simulink model "assignment_1"  (R2023b)
settings: Solver=ode3  StartTime=0.0  StopTime=Tmdl  FixedStep=To/100  RelTol=1e-3
values from neighbouring files (symbols this model uses):
  ob =     [data.mat]
undefined symbols (not defined in the file or in its folder): k_sensor, spl, T_sensor, To
libraries: fl_lib x33, nesl_utility x27
settings Model: Creator=deniskirbaba  LastModifiedBy=deniskirbaba

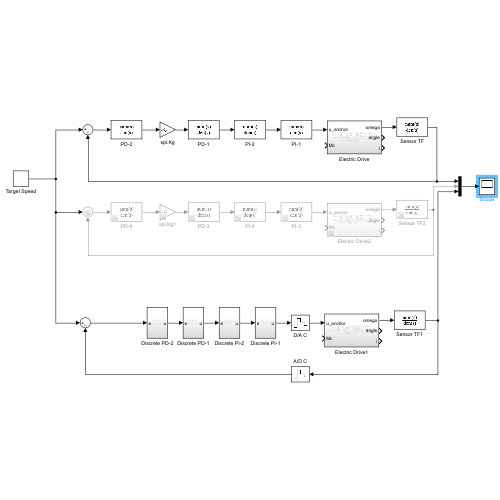
[thumbnail: Simulink's stored preview of the top-level diagram]
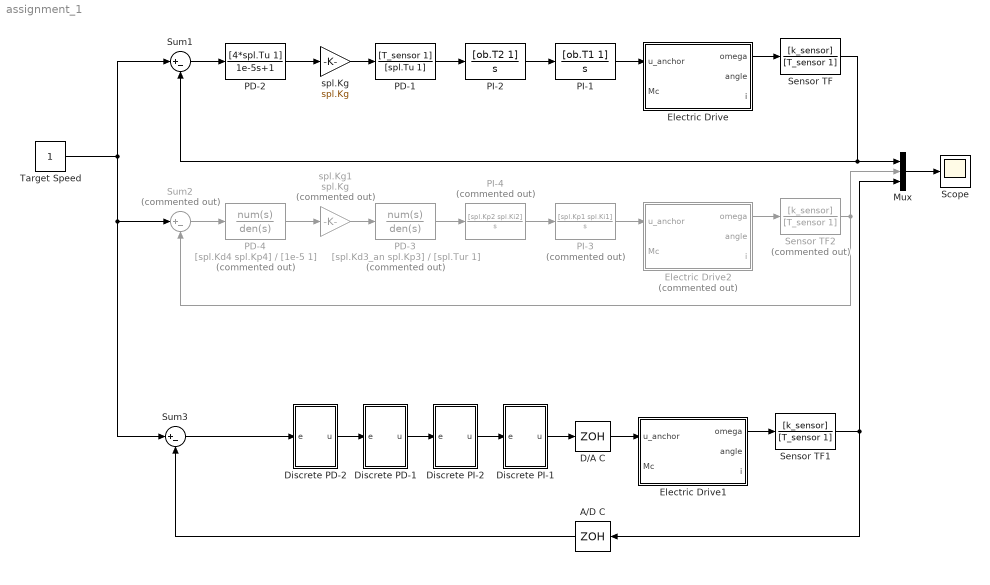
== system assignment_1 ==
  A/D C : ZeroOrderHold  SampleTime=To
  D/A C : ZeroOrderHold  SampleTime=To
  Discrete PD-1 : Subsystem
  Discrete PD-2 : Subsystem
  Discrete PI-1 : Subsystem
  Discrete PI-2 : Subsystem
  Electric Drive : Subsystem
  Electric Drive1 : Subsystem
  Electric Drive2 : Subsystem  Commented=on
  Mux : Mux  Inputs=3
  PD-1 : TransferFcn  Numerator=[T_sensor 1]  Denominator=[spl.Tu 1]
  PD-2 : TransferFcn  Numerator=[4*spl.Tu 1]  Denominator=[1e-5 1]
  PD-3 : TransferFcn  Commented=on  Numerator=[spl.Kd3_an spl.Kp3]  Denominator=[spl.Tur 1]
  PD-4 : TransferFcn  Commented=on  Numerator=[spl.Kd4 spl.Kp4]  Denominator=[1e-5 1]
  PI-1 : TransferFcn  Numerator=[ob.T1 1]  Denominator=[1 0]
  PI-2 : TransferFcn  Numerator=[ob.T2 1]  Denominator=[1 0]
  PI-3 : TransferFcn  Commented=on  Numerator=[spl.Kp1 spl.Ki1]  Denominator=[1 0]
  PI-4 : TransferFcn  Commented=on  Numerator=[spl.Kp2 spl.Ki2]  Denominator=[1 0]
  Scope : Scope
  Sensor TF : TransferFcn  Numerator=[k_sensor]  Denominator=[T_sensor 1]
  Sensor TF1 : TransferFcn  Numerator=[k_sensor]  Denominator=[T_sensor 1]
  Sensor TF2 : TransferFcn  Commented=on  Numerator=[k_sensor]  Denominator=[T_sensor 1]
  Sum1 : Sum  Inputs=|+-
  Sum2 : Sum  Commented=on  Inputs=|+-
  Sum3 : Sum  Inputs=|+-
  Target Speed : Constant
  spl.Kg : Gain  Gain=spl.Kg
  spl.Kg1 : Gain  Commented=on  Gain=spl.Kg
  wires:
  Electric Drive1/1(omega) -> Sensor TF1/1
  Mux/1 -> Scope/1
  D/A C/1 -> Electric Drive1/1(u_anchor)
  A/D C/1 -> Sum3/2
  Electric Drive/1(omega) -> Sensor TF/1
  Sum3/1 -> Discrete PD-2/1(e)
  Sum1/1 -> PD-2/1
  Discrete PD-1/1(u) -> Discrete PI-2/1(e)
  Sensor TF/1 -> Sum1/2, Mux/1
  Sensor TF1/1 -> A/D C/1, Mux/3
  PI-1/1 -> Electric Drive/1(u_anchor)
  PD-2/1 -> spl.Kg/1
  PI-2/1 -> PI-1/1
  PD-1/1 -> PI-2/1
  spl.Kg/1 -> PD-1/1
  Discrete PI-1/1(u) -> D/A C/1
  Discrete PI-2/1(u) -> Discrete PI-1/1(e)
  Discrete PD-2/1(u) -> Discrete PD-1/1(e)
  spl.Kg1/1 -> PD-3/1
  Electric Drive2/1(omega) -> Sensor TF2/1
  PD-3/1 -> PI-4/1
  PI-4/1 -> PI-3/1
  PD-4/1 -> spl.Kg1/1
  PI-3/1 -> Electric Drive2/1(u_anchor)
  Sum2/1 -> PD-4/1
  Target Speed/1 -> Sum1/1, Sum3/1, Sum2/1
  Sensor TF2/1 -> Sum2/2, Mux/2

== system assignment_1/Discrete PD-1 ==
  e : Inport
  D-regulator2 : Subsystem
  Sum4 : Sum  Inputs=++|
  spl.Kd3 : Gain  Gain=spl.Kd3
  spl.Kp3 : Gain  Gain=spl.Kp3
  u : Outport
  wires:
  e/1 -> spl.Kd3/1, spl.Kp3/1
  spl.Kd3/1 -> D-regulator2/1(e)
  spl.Kp3/1 -> Sum4/1
  D-regulator2/1(u) -> Sum4/2
  Sum4/1 -> u/1

== system assignment_1/Discrete PD-2 ==
  e : Inport
  D-regulator2 : Subsystem
  Sum4 : Sum  Inputs=++|
  spl.Kd4 : Gain  Gain=spl.Kd4
  spl.Kp4 : Gain  Gain=spl.Kp4
  u : Outport
  wires:
  e/1 -> spl.Kd4/1, spl.Kp4/1
  spl.Kd4/1 -> D-regulator2/1(e)
  spl.Kp4/1 -> Sum4/1
  D-regulator2/1(u) -> Sum4/2
  Sum4/1 -> u/1

== system assignment_1/Discrete PI-1 ==
  e : Inport
  Sum2 : Sum  Inputs=|++
  i trap : Subsystem
  spl.Ki1 : Gain  Gain=spl.Ki1
  spl.Kp1 : Gain  Gain=spl.Kp1
  u : Outport
  wires:
  e/1 -> spl.Ki1/1, spl.Kp1/1
  spl.Kp1/1 -> Sum2/1
  Sum2/1 -> u/1
  i trap/1(u) -> Sum2/2
  spl.Ki1/1 -> i trap/1(e)

== system assignment_1/Discrete PI-2 ==
  e : Inport
  Sum2 : Sum  Inputs=|++
  i trap : Subsystem
  spl.Ki2 : Gain  Gain=spl.Ki2
  spl.Kp2 : Gain  Gain=spl.Kp2
  u : Outport
  wires:
  e/1 -> spl.Ki2/1, spl.Kp2/1
  spl.Kp2/1 -> Sum2/1
  Sum2/1 -> u/1
  i trap/1(u) -> Sum2/2
  spl.Ki2/1 -> i trap/1(e)

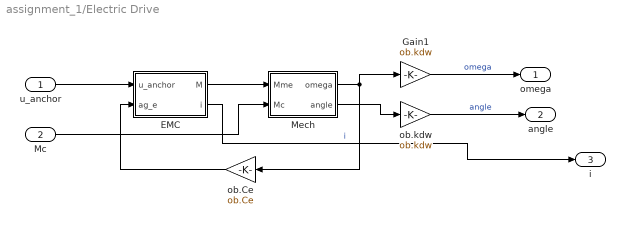
== system assignment_1/Electric Drive ==
  u_anchor : Inport
  Mc : Inport  Port=2
  EMC : Subsystem
  Gain1 : Gain  Gain=ob.kdw
  Mech : Subsystem
  ob.Ce : Gain  Gain=ob.Ce
  ob.kdw : Gain  Gain=ob.kdw
  omega : Outport
  angle : Outport  Port=2
  i : Outport  Port=3
  wires:
  Mech/1(omega) -> ob.Ce/1, Gain1/1
  Mc/1 -> Mech/2(Mc)
  Gain1/1 -> omega/1  "omega"
  EMC/1(M) -> Mech/1(Mme)
  ob.kdw/1 -> angle/1  "angle"
  Mech/2(angle) -> ob.kdw/1
  EMC/2(i) -> i/1  "i"
  ob.Ce/1 -> EMC/2(ag_e)
  u_anchor/1 -> EMC/1(u_anchor)

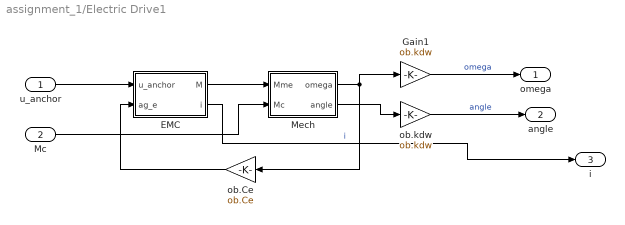
== system assignment_1/Electric Drive1 ==
  u_anchor : Inport
  Mc : Inport  Port=2
  EMC : Subsystem
  Gain1 : Gain  Gain=ob.kdw
  Mech : Subsystem
  ob.Ce : Gain  Gain=ob.Ce
  ob.kdw : Gain  Gain=ob.kdw
  omega : Outport
  angle : Outport  Port=2
  i : Outport  Port=3
  wires:
  Mech/1(omega) -> ob.Ce/1, Gain1/1
  Mc/1 -> Mech/2(Mc)
  Gain1/1 -> omega/1  "omega"
  EMC/1(M) -> Mech/1(Mme)
  ob.kdw/1 -> angle/1  "angle"
  Mech/2(angle) -> ob.kdw/1
  EMC/2(i) -> i/1  "i"
  ob.Ce/1 -> EMC/2(ag_e)
  u_anchor/1 -> EMC/1(u_anchor)

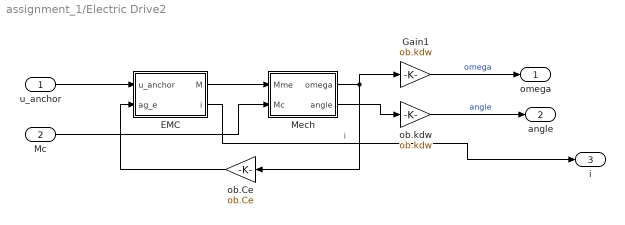
== system assignment_1/Electric Drive2 ==
  u_anchor : Inport
  Mc : Inport  Port=2
  EMC : Subsystem
  Gain1 : Gain  Gain=ob.kdw
  Mech : Subsystem
  ob.Ce : Gain  Gain=ob.Ce
  ob.kdw : Gain  Gain=ob.kdw
  omega : Outport
  angle : Outport  Port=2
  i : Outport  Port=3
  wires:
  Mech/1(omega) -> ob.Ce/1, Gain1/1
  Mc/1 -> Mech/2(Mc)
  Gain1/1 -> omega/1  "omega"
  EMC/1(M) -> Mech/1(Mme)
  ob.kdw/1 -> angle/1  "angle"
  Mech/2(angle) -> ob.kdw/1
  EMC/2(i) -> i/1  "i"
  ob.Ce/1 -> EMC/2(ag_e)
  u_anchor/1 -> EMC/1(u_anchor)

== system assignment_1/Discrete PD-1/D-regulator2 ==
  e : Inport
  Sum : Sum  Inputs=|+-
  Unit Delay : UnitDelay  SampleTime=To  HasFrameUpgradeWarning=on
  u : Outport
  wires:
  Unit Delay/1 -> Sum/2
  e/1 -> Unit Delay/1, Sum/1
  Sum/1 -> u/1

== system assignment_1/Discrete PD-2/D-regulator2 ==
  e : Inport
  Sum : Sum  Inputs=|+-
  Unit Delay : UnitDelay  SampleTime=To  HasFrameUpgradeWarning=on
  u : Outport
  wires:
  Unit Delay/1 -> Sum/2
  e/1 -> Unit Delay/1, Sum/1
  Sum/1 -> u/1

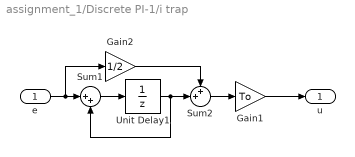
== system assignment_1/Discrete PI-1/i trap ==
  e : Inport
  Gain1 : Gain  Gain=To
  Gain2 : Gain  Gain=1/2
  Sum1 : Sum  Inputs=|++
  Sum2 : Sum  Inputs=++|
  Unit Delay1 : UnitDelay  SampleTime=To  HasFrameUpgradeWarning=on
  u : Outport
  wires:
  Unit Delay1/1 -> Sum2/2, Sum1/2
  Sum2/1 -> Gain1/1
  Gain2/1 -> Sum2/1
  Sum1/1 -> Unit Delay1/1
  e/1 -> Gain2/1, Sum1/1
  Gain1/1 -> u/1

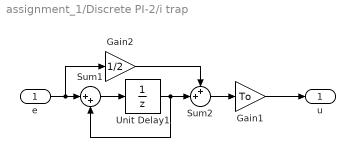
== system assignment_1/Discrete PI-2/i trap ==
  e : Inport
  Gain1 : Gain  Gain=To
  Gain2 : Gain  Gain=1/2
  Sum1 : Sum  Inputs=|++
  Sum2 : Sum  Inputs=++|
  Unit Delay1 : UnitDelay  SampleTime=To  HasFrameUpgradeWarning=on
  u : Outport
  wires:
  Unit Delay1/1 -> Sum2/2, Sum1/2
  Sum2/1 -> Gain1/1
  Gain2/1 -> Sum2/1
  Sum1/1 -> Unit Delay1/1
  e/1 -> Gain2/1, Sum1/1
  Gain1/1 -> u/1

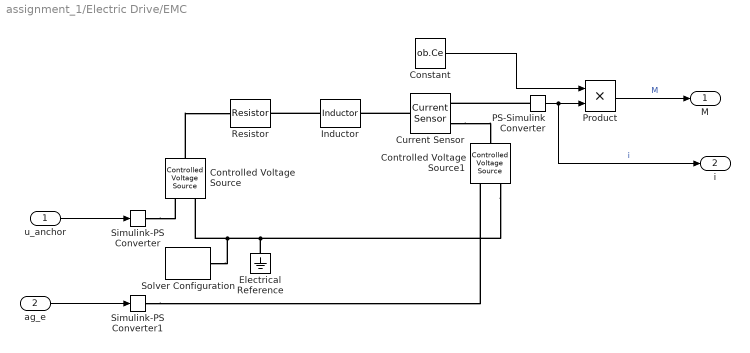
== system assignment_1/Electric Drive/EMC ==
  u_anchor : Inport
  ag_e : Inport  Port=2
  Constant : Constant  Value=ob.Ce
  Controlled Voltage Source : fl_lib/Electrical/Electrical Sources/Controlled Voltage Source
  Controlled Voltage Source1 : fl_lib/Electrical/Electrical Sources/Controlled Voltage Source
  Current Sensor : fl_lib/Electrical/Electrical Sensors/Current Sensor
  Electrical Reference : fl_lib/Electrical/Electrical Elements/Electrical Reference
  Inductor : fl_lib/Electrical/Electrical Elements/Inductor  l=ob.L H  r=0 Ohm  g=1e-9 1/Ohm  i_specify=off  i_priority=None  i=0 A  i_nominal_specify=off  i_nominal_unit=A  i_nominal_value=1  v_specify=off  v_priority=None  v=0 V  v_nominal_specify=off  v_nominal_unit=V  v_nominal_value=1  i_L_specify=off  i_L_priority=High  i_L=0 A  i_L_nominal_specify=off  i_L_nominal_unit=A  i_L_nominal_value=1
  PS-Simulink Converter : nesl_utility/PS-Simulink Converter  PhysicalDomain=network_engine_domain  SubClassName=ps_output  LeftPortType=input  RightPortType=output  PseudoPeriodic=off  Frequencies=[]  VectorFormat=inherit  Unit=inherit  AffineConversion=off
  Product : Product
  Resistor : fl_lib/Electrical/Electrical Elements/Resistor  R=ob.R Ohm  i_specify=off  i_priority=None  i=0 A  i_nominal_specify=off  i_nominal_unit=A  i_nominal_value=1  v_specify=off  v_priority=None  v=0 V  v_nominal_specify=off  v_nominal_unit=V  v_nominal_value=1
  Simulink-PS Converter : nesl_utility/Simulink-PS Converter  PhysicalDomain=network_engine_domain  SubClassName=ps_input  LeftPortType=input  RightPortType=output  PseudoPeriodic=off  Frequencies=[]  NoiseDistribution=none  NoiseParameters=[]  Unit=1  AffineConversion=off  FilteringAndDerivatives=provide  SimscapeFilterOrder=1  InputFilterTimeConstant=0.001  UdotUserProvided=0
  Simulink-PS Converter1 : nesl_utility/Simulink-PS Converter  PhysicalDomain=network_engine_domain  SubClassName=ps_input  LeftPortType=input  RightPortType=output  PseudoPeriodic=off  Frequencies=[]  NoiseDistribution=none  NoiseParameters=[]  Unit=1  AffineConversion=off  FilteringAndDerivatives=provide  SimscapeFilterOrder=1  InputFilterTimeConstant=0.001  UdotUserProvided=0
  Solver Configuration : nesl_utility/Solver Configuration  PhysicalDomain=network_engine_domain  SubClassName=solver  LeftPortType=input  RightPortType=generic  Tones=[]  Harmonics=[]  SimulateNoise=off  Profile=off  UseLocalSampling=off  EnableSwitchedLinearOptims=on  FrequencyDomain=off  UseCCode=off  RelTol=0.001  AbsTol=0.001  MinStep=1e-09  ToWorkspace=off  RevertToSquareIcSolve=off  NumHomotopyIterations=100  PhasorMode=off  PhasorModeNumHarmonics=1  ConsistencySolver=NEWTON_XTOL_AFTER_FTOL  IndexReductionMethod=DerivativeReplacement  DoDC=off  ResidualTolerance=1e-09  ConsistencyTolSource=GLOBAL  ConsistencyAbsTol=0.001  ConsistencyRelTol=0.001  ConsistencyTolFactor=0.001  UseLocalSolver=off  LocalSolverChoice=NE_BACKWARD_EULER_ADVANCER  ResolveIndetEquations=on  FunctionEvalNumThread=1  LocalSolverSampleTime=0.001  DoFixedCost=off  MaxNonlinIter=3  MaxModeIter=2  ComputeImpulses=off  ImpulseIterations=2  LinearAlgebra=auto  LinearAlgebraNumThread=0  EquationFormulation=NE_TIME_EF  DelaysMemoryBudget=1024  AutomaticFiltering=on  FilteringTimeConstant=0.001  PartitionStorageMethod=AS_NEEDED  PartitionMemoryBudget=1024  PartitionMethod=ROBUST  MultibodyUseLocalSolver=off  MultibodyLocalSolverChoice=ODE1  MultibodyLocalSolverSampleTime=0.001
  M : Outport
  i : Outport  Port=2
  wires:
  Constant/1 -> Product/1
  PS-Simulink Converter/1 -> i/1, Product/2  "i"
  ag_e/1 -> Simulink-PS Converter1/1
  Product/1 -> M/1  "M"
  u_anchor/1 -> Simulink-PS Converter/1
  connections:
  Current Sensor/LConn1 -- Inductor/RConn1
  Inductor/LConn1 -- Resistor/RConn1
  Controlled Voltage Source/LConn1 -- Resistor/LConn1
  Electrical Reference/LConn1 -- Solver Configuration/RConn1 -- Controlled Voltage Source/RConn2 -- Controlled Voltage Source1/RConn2
  PS-Simulink Converter/LConn1 -- Current Sensor/RConn1
  Current Sensor/RConn2 -- Controlled Voltage Source1/LConn1
  Simulink-PS Converter/RConn1 -- Controlled Voltage Source/RConn1
  Simulink-PS Converter1/RConn1 -- Controlled Voltage Source1/RConn1

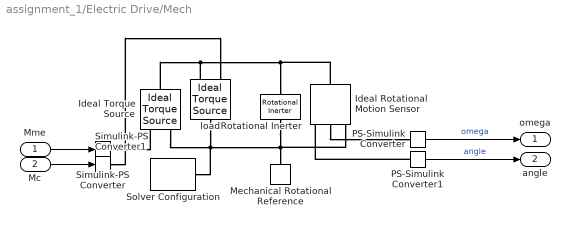
== system assignment_1/Electric Drive/Mech ==
  Mme : Inport
  Mc : Inport  Port=2
  Ideal Rotational Motion Sensor : fl_lib/Mechanical/Mechanical Sensors/Ideal Rotational Motion Sensor  reference=foundation.enum.MeasurementReference.difference  acceleration_port=false  velocity_port=true  position_port=true  wrap_angle=false  offset=0 rad
  Ideal Torque Source : fl_lib/Mechanical/Mechanical Sources/Ideal Torque Source
  Mechanical Rotational Reference : fl_lib/Mechanical/Rotational Elements/Mechanical Rotational Reference
  PS-Simulink Converter : nesl_utility/PS-Simulink Converter  PhysicalDomain=network_engine_domain  SubClassName=ps_output  LeftPortType=input  RightPortType=output  PseudoPeriodic=off  Frequencies=[]  VectorFormat=inherit  Unit=inherit  AffineConversion=off
  PS-Simulink Converter1 : nesl_utility/PS-Simulink Converter  PhysicalDomain=network_engine_domain  SubClassName=ps_output  LeftPortType=input  RightPortType=output  PseudoPeriodic=off  Frequencies=[]  VectorFormat=inherit  Unit=inherit  AffineConversion=off
  Rotational Inerter : fl_lib/Mechanical/Rotational Elements/Rotational Inerter  B=ob.J kg*m^2  w_specify=off  w_priority=High  w=0 rad/s  w_nominal_specify=off  w_nominal_unit=rad/s  w_nominal_value=1  t_specify=off  t_priority=None  t=0 N*m  t_nominal_specify=off  t_nominal_unit=N*m  t_nominal_value=1
      settings: InternalSimscapePortConfiguration="{\"Bottom\":[],\"Left\":[{\"id\":\"R\",\"label\":\"R\",\"type\":\"foundation.mechanical.rotational.rotational\"}],\"Right\":[{\"id\":\"C\",\"label\":\"C\",\"type\":\"foundation.mechanical.rotational.rotational\"}],\"Top\":[]}"
  Simulink-PS Converter : nesl_utility/Simulink-PS Converter  PhysicalDomain=network_engine_domain  SubClassName=ps_input  LeftPortType=input  RightPortType=output  PseudoPeriodic=off  Frequencies=[]  NoiseDistribution=none  NoiseParameters=[]  Unit=1  AffineConversion=off  FilteringAndDerivatives=provide  SimscapeFilterOrder=1  InputFilterTimeConstant=0.001  UdotUserProvided=0
  Simulink-PS Converter1 : nesl_utility/Simulink-PS Converter  PhysicalDomain=network_engine_domain  SubClassName=ps_input  LeftPortType=input  RightPortType=output  PseudoPeriodic=off  Frequencies=[]  NoiseDistribution=none  NoiseParameters=[]  Unit=1  AffineConversion=off  FilteringAndDerivatives=provide  SimscapeFilterOrder=1  InputFilterTimeConstant=0.001  UdotUserProvided=0
  Solver Configuration : nesl_utility/Solver Configuration  PhysicalDomain=network_engine_domain  SubClassName=solver  LeftPortType=input  RightPortType=generic  Tones=[]  Harmonics=[]  SimulateNoise=off  Profile=off  UseLocalSampling=off  EnableSwitchedLinearOptims=on  FrequencyDomain=off  UseCCode=off  RelTol=0.001  AbsTol=0.001  MinStep=1e-09  ToWorkspace=off  RevertToSquareIcSolve=off  NumHomotopyIterations=100  PhasorMode=off  PhasorModeNumHarmonics=1  ConsistencySolver=NEWTON_XTOL_AFTER_FTOL  IndexReductionMethod=DerivativeReplacement  DoDC=off  ResidualTolerance=1e-09  ConsistencyTolSource=GLOBAL  ConsistencyAbsTol=0.001  ConsistencyRelTol=0.001  ConsistencyTolFactor=0.001  UseLocalSolver=off  LocalSolverChoice=NE_BACKWARD_EULER_ADVANCER  ResolveIndetEquations=on  FunctionEvalNumThread=1  LocalSolverSampleTime=0.001  DoFixedCost=off  MaxNonlinIter=3  MaxModeIter=2  ComputeImpulses=off  ImpulseIterations=2  LinearAlgebra=auto  LinearAlgebraNumThread=0  EquationFormulation=NE_TIME_EF  DelaysMemoryBudget=1024  AutomaticFiltering=on  FilteringTimeConstant=0.001  PartitionStorageMethod=AS_NEEDED  PartitionMemoryBudget=1024  PartitionMethod=ROBUST  MultibodyUseLocalSolver=off  MultibodyLocalSolverChoice=ODE1  MultibodyLocalSolverSampleTime=0.001
  load : fl_lib/Mechanical/Mechanical Sources/Ideal Torque Source
  omega : Outport
  angle : Outport  Port=2
  wires:
  PS-Simulink Converter/1 -> omega/1  "omega"
  Mme/1 -> Simulink-PS Converter/1
  Mc/1 -> Simulink-PS Converter1/1
  PS-Simulink Converter1/1 -> angle/1  "angle"
  connections:
  PS-Simulink Converter1/LConn1 -- Ideal Rotational Motion Sensor/RConn3
  Ideal Torque Source/RConn2 -- Solver Configuration/RConn1 -- load/LConn1 -- Mechanical Rotational Reference/LConn1 -- Rotational Inerter/RConn1 -- Ideal Rotational Motion Sensor/RConn1
  Ideal Torque Source/LConn1 -- load/RConn2 -- Rotational Inerter/LConn1 -- Ideal Rotational Motion Sensor/LConn1
  Simulink-PS Converter1/RConn1 -- load/RConn1
  Ideal Rotational Motion Sensor/RConn2 -- PS-Simulink Converter/LConn1
  Simulink-PS Converter/RConn1 -- Ideal Torque Source/RConn1

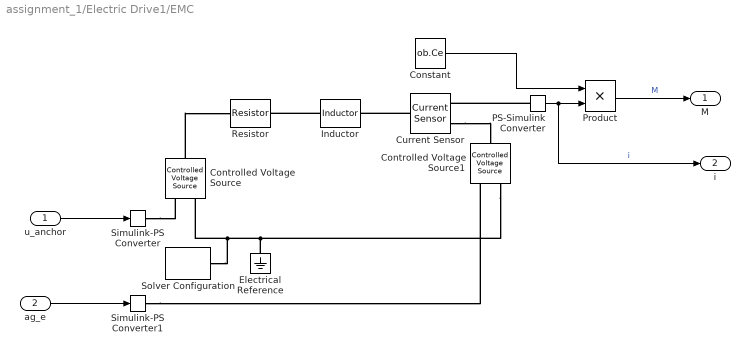
== system assignment_1/Electric Drive1/EMC ==
  u_anchor : Inport
  ag_e : Inport  Port=2
  Constant : Constant  Value=ob.Ce
  Controlled Voltage Source : fl_lib/Electrical/Electrical Sources/Controlled Voltage Source
  Controlled Voltage Source1 : fl_lib/Electrical/Electrical Sources/Controlled Voltage Source
  Current Sensor : fl_lib/Electrical/Electrical Sensors/Current Sensor
  Electrical Reference : fl_lib/Electrical/Electrical Elements/Electrical Reference
  Inductor : fl_lib/Electrical/Electrical Elements/Inductor  l=ob.L H  r=0 Ohm  g=1e-9 1/Ohm  i_specify=off  i_priority=None  i=0 A  i_nominal_specify=off  i_nominal_unit=A  i_nominal_value=1  v_specify=off  v_priority=None  v=0 V  v_nominal_specify=off  v_nominal_unit=V  v_nominal_value=1  i_L_specify=off  i_L_priority=High  i_L=0 A  i_L_nominal_specify=off  i_L_nominal_unit=A  i_L_nominal_value=1
  PS-Simulink Converter : nesl_utility/PS-Simulink Converter  PhysicalDomain=network_engine_domain  SubClassName=ps_output  LeftPortType=input  RightPortType=output  PseudoPeriodic=off  Frequencies=[]  VectorFormat=inherit  Unit=inherit  AffineConversion=off
  Product : Product
  Resistor : fl_lib/Electrical/Electrical Elements/Resistor  R=ob.R Ohm  i_specify=off  i_priority=None  i=0 A  i_nominal_specify=off  i_nominal_unit=A  i_nominal_value=1  v_specify=off  v_priority=None  v=0 V  v_nominal_specify=off  v_nominal_unit=V  v_nominal_value=1
  Simulink-PS Converter : nesl_utility/Simulink-PS Converter  PhysicalDomain=network_engine_domain  SubClassName=ps_input  LeftPortType=input  RightPortType=output  PseudoPeriodic=off  Frequencies=[]  NoiseDistribution=none  NoiseParameters=[]  Unit=1  AffineConversion=off  FilteringAndDerivatives=provide  SimscapeFilterOrder=1  InputFilterTimeConstant=0.001  UdotUserProvided=0
  Simulink-PS Converter1 : nesl_utility/Simulink-PS Converter  PhysicalDomain=network_engine_domain  SubClassName=ps_input  LeftPortType=input  RightPortType=output  PseudoPeriodic=off  Frequencies=[]  NoiseDistribution=none  NoiseParameters=[]  Unit=1  AffineConversion=off  FilteringAndDerivatives=provide  SimscapeFilterOrder=1  InputFilterTimeConstant=0.001  UdotUserProvided=0
  Solver Configuration : nesl_utility/Solver Configuration  PhysicalDomain=network_engine_domain  SubClassName=solver  LeftPortType=input  RightPortType=generic  Tones=[]  Harmonics=[]  SimulateNoise=off  Profile=off  UseLocalSampling=off  EnableSwitchedLinearOptims=on  FrequencyDomain=off  UseCCode=off  RelTol=0.001  AbsTol=0.001  MinStep=1e-09  ToWorkspace=off  RevertToSquareIcSolve=off  NumHomotopyIterations=100  PhasorMode=off  PhasorModeNumHarmonics=1  ConsistencySolver=NEWTON_XTOL_AFTER_FTOL  IndexReductionMethod=DerivativeReplacement  DoDC=off  ResidualTolerance=1e-09  ConsistencyTolSource=GLOBAL  ConsistencyAbsTol=0.001  ConsistencyRelTol=0.001  ConsistencyTolFactor=0.001  UseLocalSolver=off  LocalSolverChoice=NE_BACKWARD_EULER_ADVANCER  ResolveIndetEquations=on  FunctionEvalNumThread=1  LocalSolverSampleTime=0.001  DoFixedCost=off  MaxNonlinIter=3  MaxModeIter=2  ComputeImpulses=off  ImpulseIterations=2  LinearAlgebra=auto  LinearAlgebraNumThread=0  EquationFormulation=NE_TIME_EF  DelaysMemoryBudget=1024  AutomaticFiltering=on  FilteringTimeConstant=0.001  PartitionStorageMethod=AS_NEEDED  PartitionMemoryBudget=1024  PartitionMethod=ROBUST  MultibodyUseLocalSolver=off  MultibodyLocalSolverChoice=ODE1  MultibodyLocalSolverSampleTime=0.001
  M : Outport
  i : Outport  Port=2
  wires:
  Constant/1 -> Product/1
  PS-Simulink Converter/1 -> i/1, Product/2  "i"
  ag_e/1 -> Simulink-PS Converter1/1
  Product/1 -> M/1  "M"
  u_anchor/1 -> Simulink-PS Converter/1
  connections:
  Current Sensor/LConn1 -- Inductor/RConn1
  Inductor/LConn1 -- Resistor/RConn1
  Controlled Voltage Source/LConn1 -- Resistor/LConn1
  Electrical Reference/LConn1 -- Solver Configuration/RConn1 -- Controlled Voltage Source/RConn2 -- Controlled Voltage Source1/RConn2
  PS-Simulink Converter/LConn1 -- Current Sensor/RConn1
  Current Sensor/RConn2 -- Controlled Voltage Source1/LConn1
  Simulink-PS Converter/RConn1 -- Controlled Voltage Source/RConn1
  Simulink-PS Converter1/RConn1 -- Controlled Voltage Source1/RConn1

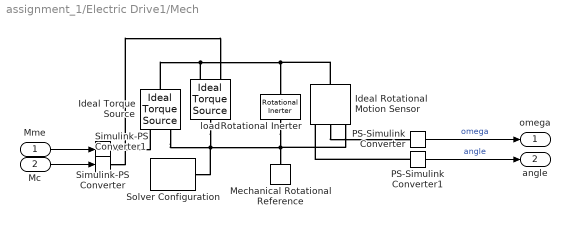
== system assignment_1/Electric Drive1/Mech ==
  Mme : Inport
  Mc : Inport  Port=2
  Ideal Rotational Motion Sensor : fl_lib/Mechanical/Mechanical Sensors/Ideal Rotational Motion Sensor  reference=foundation.enum.MeasurementReference.difference  acceleration_port=false  velocity_port=true  position_port=true  wrap_angle=false  offset=0 rad
  Ideal Torque Source : fl_lib/Mechanical/Mechanical Sources/Ideal Torque Source
  Mechanical Rotational Reference : fl_lib/Mechanical/Rotational Elements/Mechanical Rotational Reference
  PS-Simulink Converter : nesl_utility/PS-Simulink Converter  PhysicalDomain=network_engine_domain  SubClassName=ps_output  LeftPortType=input  RightPortType=output  PseudoPeriodic=off  Frequencies=[]  VectorFormat=inherit  Unit=inherit  AffineConversion=off
  PS-Simulink Converter1 : nesl_utility/PS-Simulink Converter  PhysicalDomain=network_engine_domain  SubClassName=ps_output  LeftPortType=input  RightPortType=output  PseudoPeriodic=off  Frequencies=[]  VectorFormat=inherit  Unit=inherit  AffineConversion=off
  Rotational Inerter : fl_lib/Mechanical/Rotational Elements/Rotational Inerter  B=ob.J kg*m^2  w_specify=off  w_priority=High  w=0 rad/s  w_nominal_specify=off  w_nominal_unit=rad/s  w_nominal_value=1  t_specify=off  t_priority=None  t=0 N*m  t_nominal_specify=off  t_nominal_unit=N*m  t_nominal_value=1
      settings: InternalSimscapePortConfiguration="{\"Bottom\":[],\"Left\":[{\"id\":\"R\",\"label\":\"R\",\"type\":\"foundation.mechanical.rotational.rotational\"}],\"Right\":[{\"id\":\"C\",\"label\":\"C\",\"type\":\"foundation.mechanical.rotational.rotational\"}],\"Top\":[]}"
  Simulink-PS Converter : nesl_utility/Simulink-PS Converter  PhysicalDomain=network_engine_domain  SubClassName=ps_input  LeftPortType=input  RightPortType=output  PseudoPeriodic=off  Frequencies=[]  NoiseDistribution=none  NoiseParameters=[]  Unit=1  AffineConversion=off  FilteringAndDerivatives=provide  SimscapeFilterOrder=1  InputFilterTimeConstant=0.001  UdotUserProvided=0
  Simulink-PS Converter1 : nesl_utility/Simulink-PS Converter  PhysicalDomain=network_engine_domain  SubClassName=ps_input  LeftPortType=input  RightPortType=output  PseudoPeriodic=off  Frequencies=[]  NoiseDistribution=none  NoiseParameters=[]  Unit=1  AffineConversion=off  FilteringAndDerivatives=provide  SimscapeFilterOrder=1  InputFilterTimeConstant=0.001  UdotUserProvided=0
  Solver Configuration : nesl_utility/Solver Configuration  PhysicalDomain=network_engine_domain  SubClassName=solver  LeftPortType=input  RightPortType=generic  Tones=[]  Harmonics=[]  SimulateNoise=off  Profile=off  UseLocalSampling=off  EnableSwitchedLinearOptims=on  FrequencyDomain=off  UseCCode=off  RelTol=0.001  AbsTol=0.001  MinStep=1e-09  ToWorkspace=off  RevertToSquareIcSolve=off  NumHomotopyIterations=100  PhasorMode=off  PhasorModeNumHarmonics=1  ConsistencySolver=NEWTON_XTOL_AFTER_FTOL  IndexReductionMethod=DerivativeReplacement  DoDC=off  ResidualTolerance=1e-09  ConsistencyTolSource=GLOBAL  ConsistencyAbsTol=0.001  ConsistencyRelTol=0.001  ConsistencyTolFactor=0.001  UseLocalSolver=off  LocalSolverChoice=NE_BACKWARD_EULER_ADVANCER  ResolveIndetEquations=on  FunctionEvalNumThread=1  LocalSolverSampleTime=0.001  DoFixedCost=off  MaxNonlinIter=3  MaxModeIter=2  ComputeImpulses=off  ImpulseIterations=2  LinearAlgebra=auto  LinearAlgebraNumThread=0  EquationFormulation=NE_TIME_EF  DelaysMemoryBudget=1024  AutomaticFiltering=on  FilteringTimeConstant=0.001  PartitionStorageMethod=AS_NEEDED  PartitionMemoryBudget=1024  PartitionMethod=ROBUST  MultibodyUseLocalSolver=off  MultibodyLocalSolverChoice=ODE1  MultibodyLocalSolverSampleTime=0.001
  load : fl_lib/Mechanical/Mechanical Sources/Ideal Torque Source
  omega : Outport
  angle : Outport  Port=2
  wires:
  PS-Simulink Converter/1 -> omega/1  "omega"
  Mme/1 -> Simulink-PS Converter/1
  Mc/1 -> Simulink-PS Converter1/1
  PS-Simulink Converter1/1 -> angle/1  "angle"
  connections:
  PS-Simulink Converter1/LConn1 -- Ideal Rotational Motion Sensor/RConn3
  Ideal Torque Source/RConn2 -- Solver Configuration/RConn1 -- load/LConn1 -- Mechanical Rotational Reference/LConn1 -- Rotational Inerter/RConn1 -- Ideal Rotational Motion Sensor/RConn1
  Ideal Torque Source/LConn1 -- load/RConn2 -- Rotational Inerter/LConn1 -- Ideal Rotational Motion Sensor/LConn1
  Simulink-PS Converter1/RConn1 -- load/RConn1
  Ideal Rotational Motion Sensor/RConn2 -- PS-Simulink Converter/LConn1
  Simulink-PS Converter/RConn1 -- Ideal Torque Source/RConn1

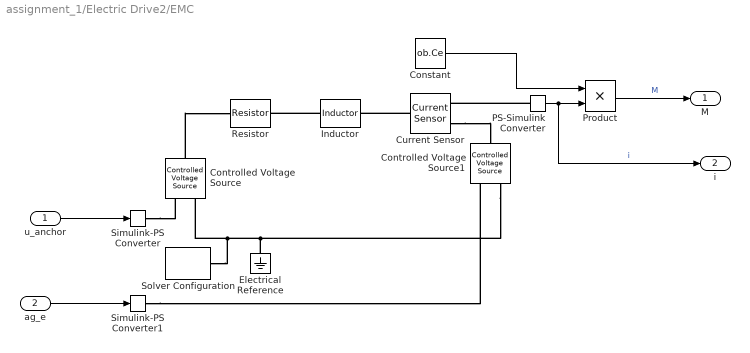
== system assignment_1/Electric Drive2/EMC ==
  u_anchor : Inport
  ag_e : Inport  Port=2
  Constant : Constant  Value=ob.Ce
  Controlled Voltage Source : fl_lib/Electrical/Electrical Sources/Controlled Voltage Source
  Controlled Voltage Source1 : fl_lib/Electrical/Electrical Sources/Controlled Voltage Source
  Current Sensor : fl_lib/Electrical/Electrical Sensors/Current Sensor
  Electrical Reference : fl_lib/Electrical/Electrical Elements/Electrical Reference
  Inductor : fl_lib/Electrical/Electrical Elements/Inductor  l=ob.L H  r=0 Ohm  g=1e-9 1/Ohm  i_specify=off  i_priority=None  i=0 A  i_nominal_specify=off  i_nominal_unit=A  i_nominal_value=1  v_specify=off  v_priority=None  v=0 V  v_nominal_specify=off  v_nominal_unit=V  v_nominal_value=1  i_L_specify=off  i_L_priority=High  i_L=0 A  i_L_nominal_specify=off  i_L_nominal_unit=A  i_L_nominal_value=1
  PS-Simulink Converter : nesl_utility/PS-Simulink Converter  PhysicalDomain=network_engine_domain  SubClassName=ps_output  LeftPortType=input  RightPortType=output  PseudoPeriodic=off  Frequencies=[]  VectorFormat=inherit  Unit=inherit  AffineConversion=off
  Product : Product
  Resistor : fl_lib/Electrical/Electrical Elements/Resistor  R=ob.R Ohm  i_specify=off  i_priority=None  i=0 A  i_nominal_specify=off  i_nominal_unit=A  i_nominal_value=1  v_specify=off  v_priority=None  v=0 V  v_nominal_specify=off  v_nominal_unit=V  v_nominal_value=1
  Simulink-PS Converter : nesl_utility/Simulink-PS Converter  PhysicalDomain=network_engine_domain  SubClassName=ps_input  LeftPortType=input  RightPortType=output  PseudoPeriodic=off  Frequencies=[]  NoiseDistribution=none  NoiseParameters=[]  Unit=1  AffineConversion=off  FilteringAndDerivatives=provide  SimscapeFilterOrder=1  InputFilterTimeConstant=0.001  UdotUserProvided=0
  Simulink-PS Converter1 : nesl_utility/Simulink-PS Converter  PhysicalDomain=network_engine_domain  SubClassName=ps_input  LeftPortType=input  RightPortType=output  PseudoPeriodic=off  Frequencies=[]  NoiseDistribution=none  NoiseParameters=[]  Unit=1  AffineConversion=off  FilteringAndDerivatives=provide  SimscapeFilterOrder=1  InputFilterTimeConstant=0.001  UdotUserProvided=0
  Solver Configuration : nesl_utility/Solver Configuration  PhysicalDomain=network_engine_domain  SubClassName=solver  LeftPortType=input  RightPortType=generic  Tones=[]  Harmonics=[]  SimulateNoise=off  Profile=off  UseLocalSampling=off  EnableSwitchedLinearOptims=on  FrequencyDomain=off  UseCCode=off  RelTol=0.001  AbsTol=0.001  MinStep=1e-09  ToWorkspace=off  RevertToSquareIcSolve=off  NumHomotopyIterations=100  PhasorMode=off  PhasorModeNumHarmonics=1  ConsistencySolver=NEWTON_XTOL_AFTER_FTOL  IndexReductionMethod=DerivativeReplacement  DoDC=off  ResidualTolerance=1e-09  ConsistencyTolSource=GLOBAL  ConsistencyAbsTol=0.001  ConsistencyRelTol=0.001  ConsistencyTolFactor=0.001  UseLocalSolver=off  LocalSolverChoice=NE_BACKWARD_EULER_ADVANCER  ResolveIndetEquations=on  FunctionEvalNumThread=1  LocalSolverSampleTime=0.001  DoFixedCost=off  MaxNonlinIter=3  MaxModeIter=2  ComputeImpulses=off  ImpulseIterations=2  LinearAlgebra=auto  LinearAlgebraNumThread=0  EquationFormulation=NE_TIME_EF  DelaysMemoryBudget=1024  AutomaticFiltering=on  FilteringTimeConstant=0.001  PartitionStorageMethod=AS_NEEDED  PartitionMemoryBudget=1024  PartitionMethod=ROBUST  MultibodyUseLocalSolver=off  MultibodyLocalSolverChoice=ODE1  MultibodyLocalSolverSampleTime=0.001
  M : Outport
  i : Outport  Port=2
  wires:
  Constant/1 -> Product/1
  PS-Simulink Converter/1 -> i/1, Product/2  "i"
  ag_e/1 -> Simulink-PS Converter1/1
  Product/1 -> M/1  "M"
  u_anchor/1 -> Simulink-PS Converter/1
  connections:
  Current Sensor/LConn1 -- Inductor/RConn1
  Inductor/LConn1 -- Resistor/RConn1
  Controlled Voltage Source/LConn1 -- Resistor/LConn1
  Electrical Reference/LConn1 -- Solver Configuration/RConn1 -- Controlled Voltage Source/RConn2 -- Controlled Voltage Source1/RConn2
  PS-Simulink Converter/LConn1 -- Current Sensor/RConn1
  Current Sensor/RConn2 -- Controlled Voltage Source1/LConn1
  Simulink-PS Converter/RConn1 -- Controlled Voltage Source/RConn1
  Simulink-PS Converter1/RConn1 -- Controlled Voltage Source1/RConn1

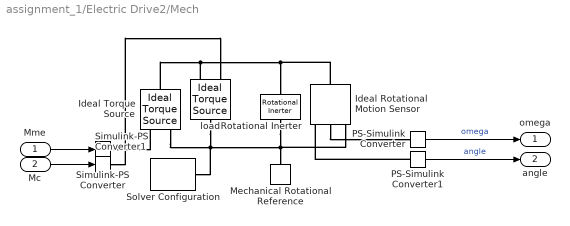
== system assignment_1/Electric Drive2/Mech ==
  Mme : Inport
  Mc : Inport  Port=2
  Ideal Rotational Motion Sensor : fl_lib/Mechanical/Mechanical Sensors/Ideal Rotational Motion Sensor  reference=foundation.enum.MeasurementReference.difference  acceleration_port=false  velocity_port=true  position_port=true  wrap_angle=false  offset=0 rad
  Ideal Torque Source : fl_lib/Mechanical/Mechanical Sources/Ideal Torque Source
  Mechanical Rotational Reference : fl_lib/Mechanical/Rotational Elements/Mechanical Rotational Reference
  PS-Simulink Converter : nesl_utility/PS-Simulink Converter  PhysicalDomain=network_engine_domain  SubClassName=ps_output  LeftPortType=input  RightPortType=output  PseudoPeriodic=off  Frequencies=[]  VectorFormat=inherit  Unit=inherit  AffineConversion=off
  PS-Simulink Converter1 : nesl_utility/PS-Simulink Converter  PhysicalDomain=network_engine_domain  SubClassName=ps_output  LeftPortType=input  RightPortType=output  PseudoPeriodic=off  Frequencies=[]  VectorFormat=inherit  Unit=inherit  AffineConversion=off
  Rotational Inerter : fl_lib/Mechanical/Rotational Elements/Rotational Inerter  B=ob.J kg*m^2  w_specify=off  w_priority=High  w=0 rad/s  w_nominal_specify=off  w_nominal_unit=rad/s  w_nominal_value=1  t_specify=off  t_priority=None  t=0 N*m  t_nominal_specify=off  t_nominal_unit=N*m  t_nominal_value=1
      settings: InternalSimscapePortConfiguration="{\"Bottom\":[],\"Left\":[{\"id\":\"R\",\"label\":\"R\",\"type\":\"foundation.mechanical.rotational.rotational\"}],\"Right\":[{\"id\":\"C\",\"label\":\"C\",\"type\":\"foundation.mechanical.rotational.rotational\"}],\"Top\":[]}"
  Simulink-PS Converter : nesl_utility/Simulink-PS Converter  PhysicalDomain=network_engine_domain  SubClassName=ps_input  LeftPortType=input  RightPortType=output  PseudoPeriodic=off  Frequencies=[]  NoiseDistribution=none  NoiseParameters=[]  Unit=1  AffineConversion=off  FilteringAndDerivatives=provide  SimscapeFilterOrder=1  InputFilterTimeConstant=0.001  UdotUserProvided=0
  Simulink-PS Converter1 : nesl_utility/Simulink-PS Converter  PhysicalDomain=network_engine_domain  SubClassName=ps_input  LeftPortType=input  RightPortType=output  PseudoPeriodic=off  Frequencies=[]  NoiseDistribution=none  NoiseParameters=[]  Unit=1  AffineConversion=off  FilteringAndDerivatives=provide  SimscapeFilterOrder=1  InputFilterTimeConstant=0.001  UdotUserProvided=0
  Solver Configuration : nesl_utility/Solver Configuration  PhysicalDomain=network_engine_domain  SubClassName=solver  LeftPortType=input  RightPortType=generic  Tones=[]  Harmonics=[]  SimulateNoise=off  Profile=off  UseLocalSampling=off  EnableSwitchedLinearOptims=on  FrequencyDomain=off  UseCCode=off  RelTol=0.001  AbsTol=0.001  MinStep=1e-09  ToWorkspace=off  RevertToSquareIcSolve=off  NumHomotopyIterations=100  PhasorMode=off  PhasorModeNumHarmonics=1  ConsistencySolver=NEWTON_XTOL_AFTER_FTOL  IndexReductionMethod=DerivativeReplacement  DoDC=off  ResidualTolerance=1e-09  ConsistencyTolSource=GLOBAL  ConsistencyAbsTol=0.001  ConsistencyRelTol=0.001  ConsistencyTolFactor=0.001  UseLocalSolver=off  LocalSolverChoice=NE_BACKWARD_EULER_ADVANCER  ResolveIndetEquations=on  FunctionEvalNumThread=1  LocalSolverSampleTime=0.001  DoFixedCost=off  MaxNonlinIter=3  MaxModeIter=2  ComputeImpulses=off  ImpulseIterations=2  LinearAlgebra=auto  LinearAlgebraNumThread=0  EquationFormulation=NE_TIME_EF  DelaysMemoryBudget=1024  AutomaticFiltering=on  FilteringTimeConstant=0.001  PartitionStorageMethod=AS_NEEDED  PartitionMemoryBudget=1024  PartitionMethod=ROBUST  MultibodyUseLocalSolver=off  MultibodyLocalSolverChoice=ODE1  MultibodyLocalSolverSampleTime=0.001
  load : fl_lib/Mechanical/Mechanical Sources/Ideal Torque Source
  omega : Outport
  angle : Outport  Port=2
  wires:
  PS-Simulink Converter/1 -> omega/1  "omega"
  Mme/1 -> Simulink-PS Converter/1
  Mc/1 -> Simulink-PS Converter1/1
  PS-Simulink Converter1/1 -> angle/1  "angle"
  connections:
  PS-Simulink Converter1/LConn1 -- Ideal Rotational Motion Sensor/RConn3
  Ideal Torque Source/RConn2 -- Solver Configuration/RConn1 -- load/LConn1 -- Mechanical Rotational Reference/LConn1 -- Rotational Inerter/RConn1 -- Ideal Rotational Motion Sensor/RConn1
  Ideal Torque Source/LConn1 -- load/RConn2 -- Rotational Inerter/LConn1 -- Ideal Rotational Motion Sensor/LConn1
  Simulink-PS Converter1/RConn1 -- load/RConn1
  Ideal Rotational Motion Sensor/RConn2 -- PS-Simulink Converter/LConn1
  Simulink-PS Converter/RConn1 -- Ideal Torque Source/RConn1
